simulink model "UAV_dynamic_model"  (R2024a)
settings: Solver=FixedStepDiscrete  StartTime=0.0  StopTime=5  FixedStep=0.001  RelTol=1e-3
undefined symbols (not defined in the file or in its folder): Accel_Body, AngularRate_Body, Attitude_quat, DiscIntNeverNeededParam, g, inertia, mass, Position_NED, Velocity_NED
settings Model: DataDictionary=DynamicModelDict.sldd  Creator=89447  LastModifiedBy=89447
settings DataIOCC: InspectSignalLogs=on

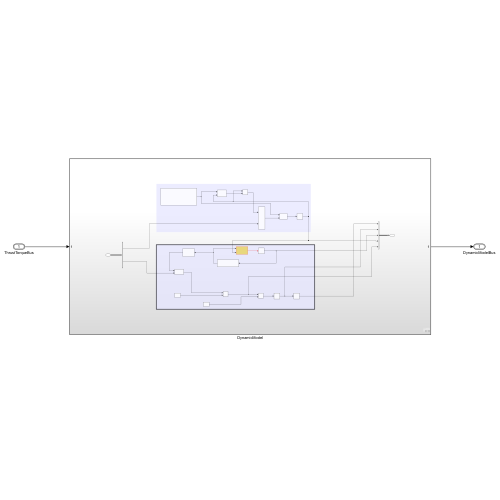
[thumbnail: Simulink's stored preview of the top-level diagram]
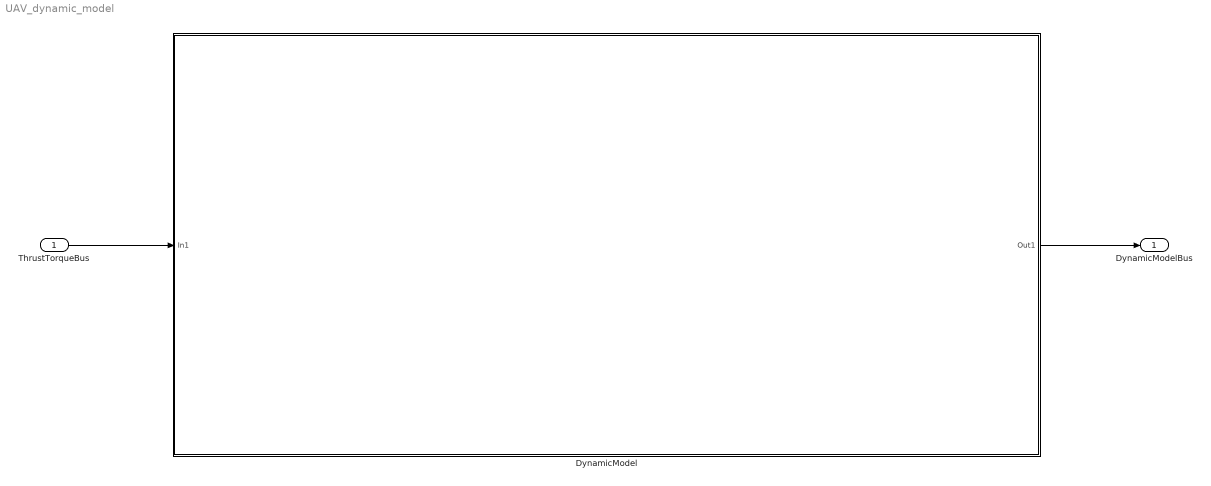
== system UAV_dynamic_model ==
  ThrustTorqueBus : Inport  OutDataTypeStr=Bus: ThrustTorqueBus
  DynamicModel : Subsystem
  DynamicModelBus : Outport  OutDataTypeStr=Bus: DynamicModelBus
  wires:
  ThrustTorqueBus/1 -> DynamicModel/1(In1)
  DynamicModel/1(Out1) -> DynamicModelBus/1

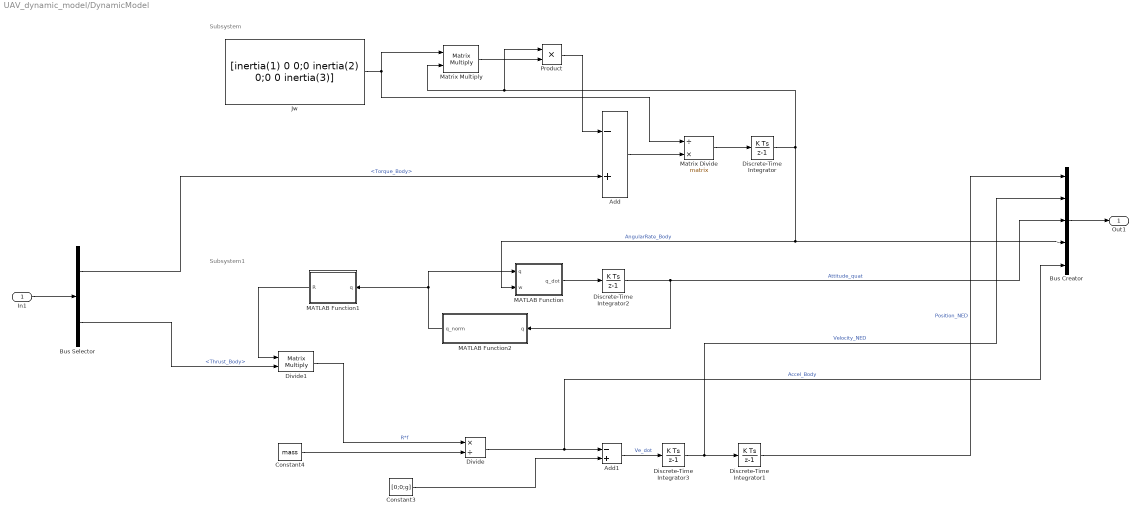
== system UAV_dynamic_model/DynamicModel ==
  note: Subsystem1
  note: Subsystem
  In1 : Inport
  Add : Sum  Inputs=-+
  Add1 : Sum  Inputs=-+
  Bus Creator : BusCreator  Inputs=Position_NED,Velocity_NED,Attitude_quat,AngularRate_Body,Accel_Body  OutDataTypeStr=Bus: DynamicModelBus  NonVirtualBus=on
  Bus Selector : BusSelector  OutputSignals=Torque_Body,Thrust_Body
  Constant3 : Constant  Value=[0;0;g]
  Constant4 : Constant  Value=mass
  Discrete-Time Integrator : DiscreteIntegrator  SampleTime=-1  ICPrevOutput=DiscIntNeverNeededParam  ICPrevScaledInput=DiscIntNeverNeededParam
  Discrete-Time Integrator1 : DiscreteIntegrator  InitialCondition=[0;0;-10]  SampleTime=-1  ICPrevOutput=DiscIntNeverNeededParam  ICPrevScaledInput=DiscIntNeverNeededParam
  Discrete-Time Integrator2 : DiscreteIntegrator  InitialCondition=[1;0;0;0]  SampleTime=-1  ICPrevOutput=DiscIntNeverNeededParam  ICPrevScaledInput=DiscIntNeverNeededParam
  Discrete-Time Integrator3 : DiscreteIntegrator  InitialCondition=[0;0;0]  SampleTime=-1  ICPrevOutput=DiscIntNeverNeededParam  ICPrevScaledInput=DiscIntNeverNeededParam
  Divide : Product  Inputs=*/
  Divide1 : Product  Inputs=**  Multiplication=Matrix(*)
  Jw : Constant  Value=[inertia(1) 0 0;0 inertia(2) 0;0 0 inertia(3)]
  MATLAB Function : MATLAB Function  TreatAsAtomicUnit=on
  MATLAB Function1 : MATLAB Function  TreatAsAtomicUnit=on
  MATLAB Function2 : MATLAB Function  TreatAsAtomicUnit=on
  Matrix Divide : Product  Inputs=/*  Multiplication=Matrix(*)
  Matrix Multiply : Product  Multiplication=Matrix(*)
  Product : Product
  Out1 : Outport
  wires:
  Discrete-Time Integrator2/1 -> Bus Creator/3, MATLAB Function2/1(q)  "Attitude_quat"
  Discrete-Time Integrator/1 -> Bus Creator/4, MATLAB Function/2(w), Matrix Multiply/2, Product/1  "AngularRate_Body"
  MATLAB Function/1(q_dot) -> Discrete-Time Integrator2/1
  Add/1 -> Matrix Divide/2
  Bus Selector/1 -> Add/2  "<Torque_Body>"
  Divide1/1 -> Divide/1  "R*f"
  Discrete-Time Integrator3/1 -> Bus Creator/2, Discrete-Time Integrator1/1  "Velocity_NED"
  Constant4/1 -> Divide/2
  Constant3/1 -> Add1/2
  Matrix Divide/1 -> Discrete-Time Integrator/1
  Bus Creator/1 -> Out1/1
  Divide/1 -> Bus Creator/5, Add1/1  "Accel_Body"
  MATLAB Function2/1(q_norm) -> MATLAB Function/1(q), MATLAB Function1/1(q)
  Add1/1 -> Discrete-Time Integrator3/1  "Ve_dot"
  MATLAB Function1/1(R) -> Divide1/1
  Matrix Multiply/1 -> Product/2
  Product/1 -> Add/1
  Jw/1 -> Matrix Divide/1, Matrix Multiply/1
  Discrete-Time Integrator1/1 -> Bus Creator/1  "Position_NED"
  Bus Selector/2 -> Divide1/2  "<Thrust_Body>"
  In1/1 -> Bus Selector/1

== matlab function UAV_dynamic_model/DynamicModel/MATLAB Function1 ==
  data: q input; R output
function R = quat2rotm(q)
% 四元数 转 旋转矩阵（3×3）
% 输入：q = [qw, qx, qy, qz]  （实部在前，Hamilton 四元数）
% 输出：R = 3×3 旋转矩阵

% 提取四元数分量
qw = q(1);
qx = q(2);
qy = q(3);
qz = q(4);

% 归一化（防止非单位四元数导致错误）
norm_q = sqrt(qw^2 + qx^2 + qy^2 + qz^2);
qw = qw / norm_q;
qx = qx / norm_q;
qy = qy / norm_q;
qz = qz / norm_q;

% 旋转矩阵公式
R = [
    1 - 2*qy^2 - 2*qz^2,     2*qx*qy - 2*qw*qz,     2*qx*qz + 2*qw*qy;
    2*qx*qy + 2*qw*qz,     1 - 2*qx^2 - 2*qz^2,     2*qy*qz - 2*qw*qx;
    2*qx*qz - 2*qw*qy,     2*qy*qz + 2*qw*qx,     1 - 2*qx^2 - 2*qy^2
    ];
end

== matlab function UAV_dynamic_model/DynamicModel/MATLAB Function2 ==
  data: q input; q_norm output
function q_norm = fcn_quat_normalize(q)
    % 输入 q 为 [4x1] 的四元数向量
    
    % 计算二范数 (模长)
    % 加上 eps (极小值) 是为了防止分母为 0 导致的计算崩溃
    n = sqrt(sum(q.^2));
    
    % 执行归一化
    q_norm = q ./ n;
end

== matlab function UAV_dynamic_model/DynamicModel/MATLAB Function ==
  data: q input; q_dot output; w input
function q_dot = fcn(q, w)
% q_dot = 1/2 * q * omega
% 输入 q: 当前四元数 [qw; qx; qy; qz] (4x1)
% 输入 w: 当前机体角速度 [p; q; r] (3x1)
% 输出 q_dot: 四元数变化率 (4x1)

% 提取角速度分量
p = w(1);
q_val = w(2); % 避免与四元数变量名 q 冲突
r = w(3);

% 构建 Omega 矩阵 (四元数微分矩阵)
% 这里的符号顺序基于 [qw, qx, qy, qz]
Omega = [ 0, -p, -q_val, -r;
          p,  0,  r,     -q_val;
          q_val, -r,  0,      p;
          r,  q_val, -p,      0 ];

% 计算导数
q_dot = 0.5 * Omega * q;

end
